simulink subsystem "Pre_Path_Planning"  (R2023b)
settings: Solver=VariableStepAuto  StartTime=0.0  StopTime=10.0  RelTol=1e-3
undefined symbols (not defined in the file): Spline_Max_Num_RefPoses, Spline_Num_Samples, Spline_Samples_Per_Pass
libraries: matrix_library x1
settings Model: Creator=FIRSTMentor  LastModifiedBy=FIRSTMentor

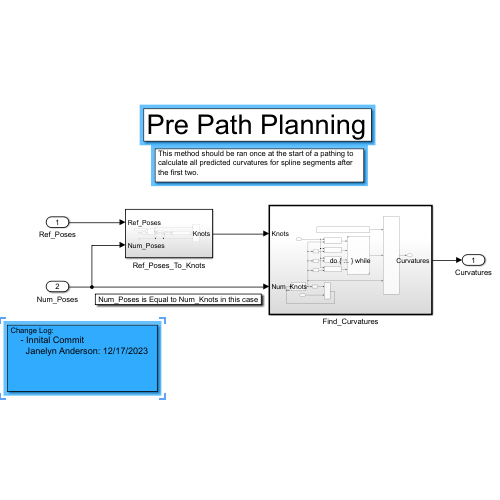
[thumbnail: Simulink's stored preview of the top-level diagram]
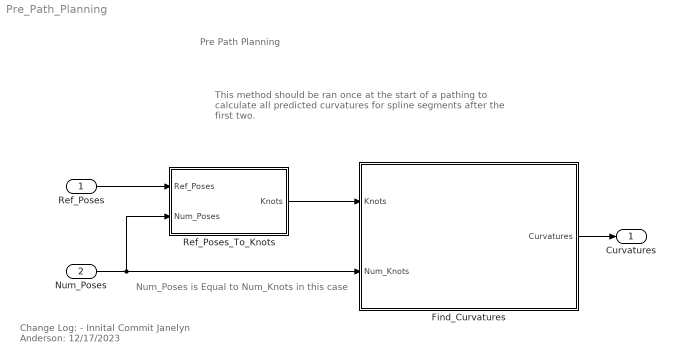
== system Pre_Path_Planning ==
  note: Num_Poses is Equal to Num_Knots in this case
  note: Pre Path Planning
  note: This method should be ran once at the start of a pathing to calculate all predicted curvatures for spline segments after the first two.
  note: Change Log:
      | - Innital Commit
      | Janelyn Anderson: 12/17/2023
  Ref_Poses : Inport  PortDimensions=[Spline_Samples_Per_Pass 3]
  Num_Poses : Inport  Port=2
  Find_Curvatures : Subsystem  TreatAsAtomicUnit=on
  Ref_Poses_To_Knots : Subsystem
  Curvatures : Outport
  wires:
  Find_Curvatures/1(Curvatures) -> Curvatures/1
  Ref_Poses/1 -> Ref_Poses_To_Knots/1(Ref_Poses)
  Ref_Poses_To_Knots/1(Knots) -> Find_Curvatures/1(Knots)
  Num_Poses/1 -> Find_Curvatures/2(Num_Knots), Ref_Poses_To_Knots/2(Num_Poses)

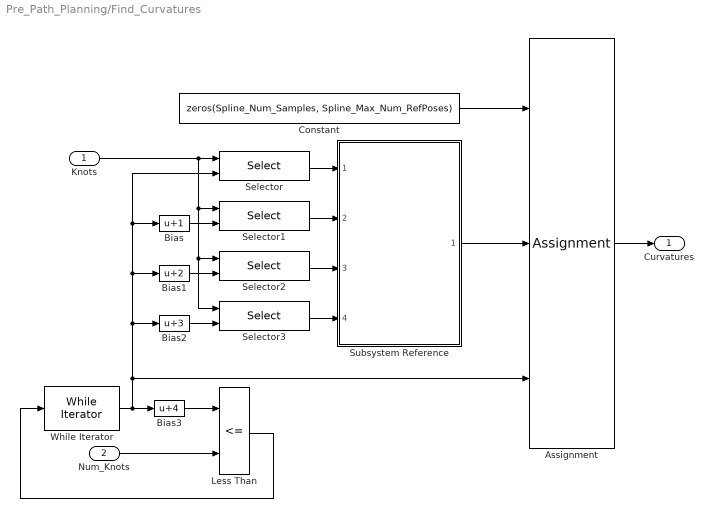
== system Pre_Path_Planning/Find_Curvatures ==
  Knots : Inport
  Num_Knots : Inport  Port=2
  Assignment : Assignment  NumberOfDimensions=2  DiagnosticForDimensions=Warning  IndexOptions=Assign all,Index vector (port)  Indices=1,1  OutputSizes=1,1
  Bias : Bias  Bias=1  SaturateOnIntegerOverflow=off
  Bias1 : Bias  Bias=2  SaturateOnIntegerOverflow=off
  Bias2 : Bias  Bias=3  SaturateOnIntegerOverflow=off
  Bias3 : Bias  Bias=4  SaturateOnIntegerOverflow=off
  Constant : Constant  Value=zeros(Spline_Num_Samples, Spline_Max_Num_RefPoses)  VectorParams1D=off
  Less Than : RelationalOperator  Operator=<=  OutDataTypeStr=boolean  RndMeth=Simplest  InputSameDT=off
  Selector{,1..3} (4 alike) : Selector  NumberOfDimensions=2  InputPortWidth=3  IndexOptions=Index vector (port),Select all  Indices=[1 3],1  OutputSizes=1,1
  Subsystem Reference : Subsystem  ReferencedSubsystem=Sample_Catmull_Rom_Curve
  While Iterator : WhileIterator  MaxIters=-1  WhileBlockType=do-while  ShowIterationPort=on
  Curvatures : Outport
  wires:
  While Iterator/1 -> Bias3/1, Assignment/3, Bias2/1, Bias1/1, Bias/1, Selector/2
  Num_Knots/1 -> Less Than/2
  Less Than/1 -> While Iterator/1
  Knots/1 -> Selector3/1, Selector2/1, Selector1/1, Selector/1
  Selector/1 -> Subsystem Reference/1
  Selector3/1 -> Subsystem Reference/4
  Selector2/1 -> Subsystem Reference/3
  Selector1/1 -> Subsystem Reference/2
  Bias2/1 -> Selector3/2
  Bias1/1 -> Selector2/2
  Bias/1 -> Selector1/2
  Bias3/1 -> Less Than/1
  Subsystem Reference/1 -> Assignment/2
  Assignment/1 -> Curvatures/1
  Constant/1 -> Assignment/1

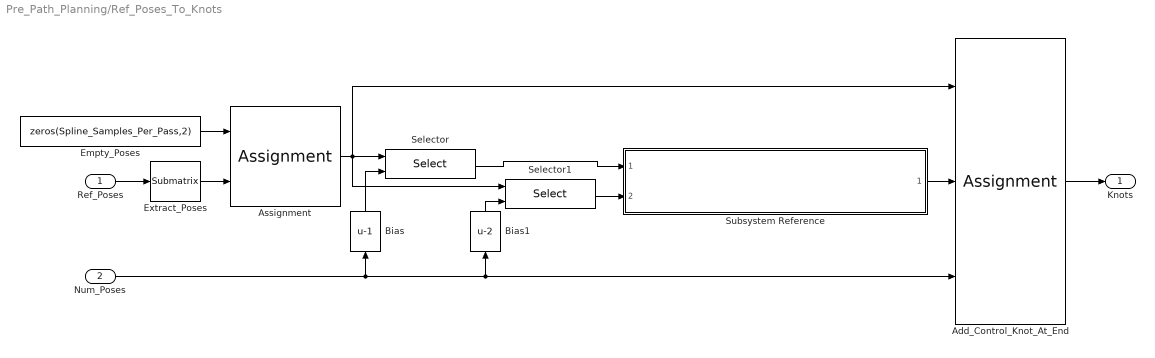
== system Pre_Path_Planning/Ref_Poses_To_Knots ==
  Ref_Poses : Inport  PortDimensions=[Spline_Samples_Per_Pass 3]
  Num_Poses : Inport  Port=2
  Add_Control_Knot_At_End : Assignment  NumberOfDimensions=2  DiagnosticForDimensions=Warning  IndexOptions=Index vector (port),Assign all  Indices=2,1  OutputSizes=1,1
  Assignment : Assignment  NumberOfDimensions=2  DiagnosticForDimensions=Warning  IndexOptions=Starting index (dialog),Assign all  Indices=1,1  OutputSizes=1,1
  Bias : Bias  Bias=-1  SaturateOnIntegerOverflow=off
  Bias1 : Bias  Bias=-2  SaturateOnIntegerOverflow=off
  Empty_Poses : Constant  Value=zeros(Spline_Samples_Per_Pass,2)
  Extract_Poses : matrix_library/Submatrix  RowSpan=Range of rows  RowStartMode=Index  RowStartIndex=2  RowEndMode=Last  RowEndIndex=1  ColSpan=Range of columns  ColStartMode=First  ColStartIndex=1  ColEndMode=Index  ColEndIndex=2
  Selector : Selector  NumberOfDimensions=2  InputPortWidth=3  IndexOptions=Index vector (port),Select all  Indices=[1 3],1  OutputSizes=1,1
  Selector1 : Selector  NumberOfDimensions=2  InputPortWidth=3  IndexOptions=Index vector (port),Select all  Indices=[1 3],1  OutputSizes=1,1
  Subsystem Reference : Subsystem  ReferencedSubsystem=Find_Control_Pose
  Knots : Outport
  wires:
  Empty_Poses/1 -> Assignment/1
  Ref_Poses/1 -> Extract_Poses/1
  Extract_Poses/1 -> Assignment/2
  Add_Control_Knot_At_End/1 -> Knots/1
  Subsystem Reference/1 -> Add_Control_Knot_At_End/2
  Selector/1 -> Subsystem Reference/1
  Selector1/1 -> Subsystem Reference/2
  Assignment/1 -> Selector/1, Add_Control_Knot_At_End/1, Selector1/1
  Num_Poses/1 -> Bias1/1, Add_Control_Knot_At_End/3, Bias/1
  Bias/1 -> Selector/2
  Bias1/1 -> Selector1/2
